simulink model "Ex1_4"  (R2015b)
settings: Solver=VariableStepAuto  StartTime=0.0  StopTime=10  RelTol=1e-3
settings Model: Creator=Mans  LastModifiedBy=Mans

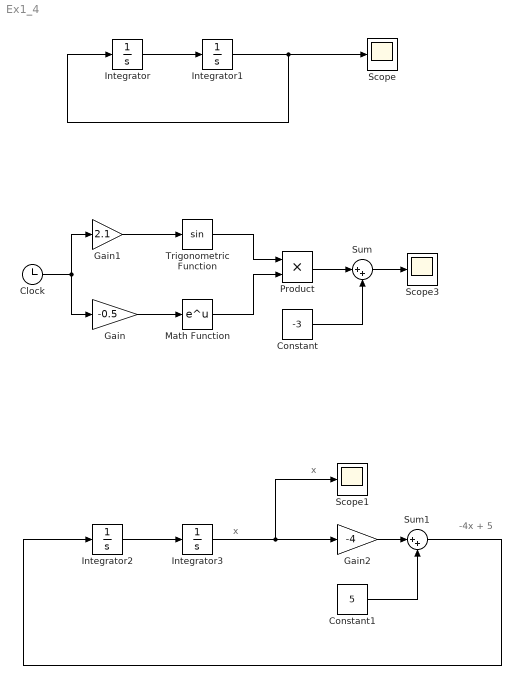
== system Ex1_4 ==
  note: -4x + 5
  note: x
  note: x
  Clock : Clock
  Constant : Constant  Value=-3
  Constant1 : Constant  Value=5
  Gain : Gain  Gain=-0.5
  Gain1 : Gain  Gain=2.1
  Gain2 : Gain  Gain=-4
  Integrator{,1..3} (4 alike) : Integrator
  Math Function : Math  SaturateOnIntegerOverflow=on
  Product : Product
  Scope : Scope
  Scope1 : Scope
  Scope3 : Scope
  Sum : Sum  Inputs=|++
  Sum1 : Sum  Inputs=|++
  Trigonometric Function : Trigonometry
  wires:
  Clock/1 -> Gain1/1, Gain/1
  Gain/1 -> Math Function/1
  Gain1/1 -> Trigonometric Function/1
  Trigonometric Function/1 -> Product/1
  Math Function/1 -> Product/2
  Product/1 -> Sum/1
  Constant/1 -> Sum/2
  Sum/1 -> Scope3/1
  Integrator/1 -> Integrator1/1
  Integrator1/1 -> Scope/1, Integrator/1
  Integrator2/1 -> Integrator3/1
  Integrator3/1 -> Scope1/1, Gain2/1
  Gain2/1 -> Sum1/1
  Constant1/1 -> Sum1/2
  Sum1/1 -> Integrator2/1
